simulink model "Square_PWM"  (R2019a)
settings: Solver=VariableStepAuto  StartTime=0.0  StopTime=0.2  RelTol=1e-3
libraries: powerlib x15, simulink x1, powerlib_meascontrol x1
settings Model: Creator=omar_  LastModifiedBy=omar_
settings DataIOCC: ReturnWorkspaceOutputs=off

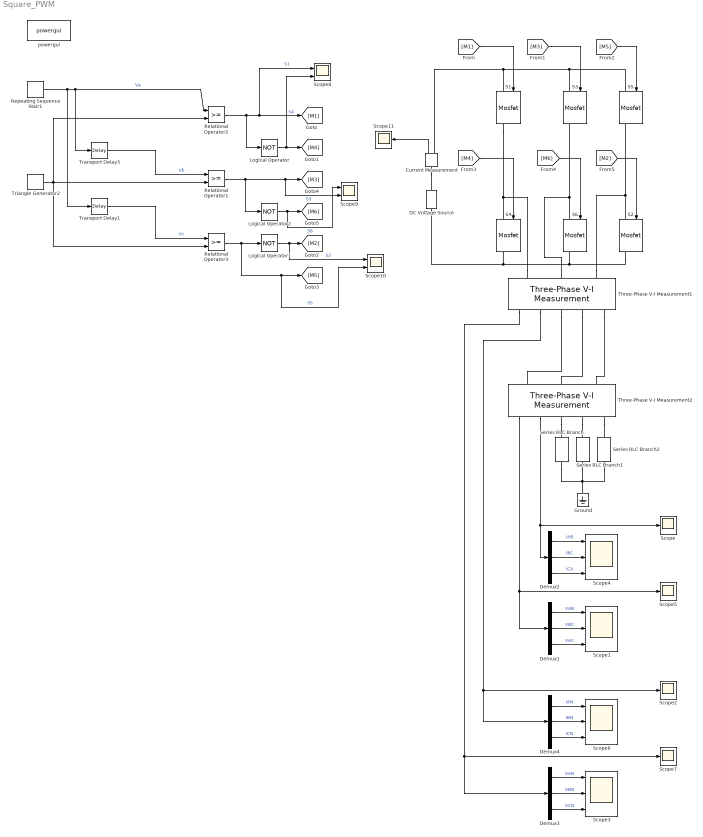
== system Square_PWM ==
  Current Measurement : powerlib/Measurements/Current Measurement  PhasorSimulation=off  OutputType=Complex  PSBequivalent=0
      settings: SourceProductName=Simscape Electrical
  DC Voltage Source : powerlib/Electrical Sources/DC Voltage Source  Amplitude=100  Measurements=None
      settings: SourceProductName=Simscape Electrical
  Demux{1..4} (4 alike) : Demux  Outputs=3
  Ground : powerlib/Elements/Ground  LConnTagsString=a
      settings: SourceProductName=Simscape Electrical
  Logical Operator : Logic  Operator=NOT  AllPortsSameDT=off  OutDataTypeStr=boolean
  Logical Operator1 : Logic  Operator=NOT  AllPortsSameDT=off  OutDataTypeStr=boolean
  Logical Operator2 : Logic  Operator=NOT  AllPortsSameDT=off  OutDataTypeStr=boolean
  Relational Operator1 : RelationalOperator  OutDataTypeStr=boolean  RndMeth=Simplest
  Relational Operator2 : RelationalOperator  OutDataTypeStr=boolean  RndMeth=Simplest
  Relational Operator3 : RelationalOperator  OutDataTypeStr=boolean  RndMeth=Simplest
  Repeating Sequence Stair1 : simulink/Sources/Repeating Sequence Stair  OutValues=[0.707, 0.707, -0.707, -0.707].'  tsamp=0.005  OutMin=[]  OutMax=[]  OutDataTypeStr=double  OutputDataTypeScalingMode=double  OutDataType=fixdt(0,8)  ConRadixGroup=Best Precision: Vector-wise  OutScaling=2^-12
  S{1..6} (6 alike) : powerlib/Power Electronics/Mosfet  Ron=0  Lon=0  Rd=0  Vfd=0  IC=0  Rs=1e5  Cs=inf  Measurements=on
      settings: SourceProductName=Simscape Electrical
  Scope{,2,5,7,11} (5 alike) : Scope
  Scope{1,3..4,6} (4 alike) : Scope  NumInputPorts=3
  Scope10 : Scope  NumInputPorts=2
  Scope8 : Scope  NumInputPorts=2
  Scope9 : Scope  NumInputPorts=2
  Series RLC Branch : powerlib/Elements/Series RLC Branch  LConnTagsString=__new0  RConnTagsString=__new0  BranchType=RL  Resistance=1  Inductance=5e-3  SetiL0=off  InitialCurrent=0  Capacitance=1e-6  Setx0=off  InitialVoltage=0  Measurements=None
      settings: SourceProductName=Simscape Electrical
  Series RLC Branch1 : powerlib/Elements/Series RLC Branch  LConnTagsString=__new0  RConnTagsString=__new0  BranchType=RL  Resistance=1  Inductance=5e-3  SetiL0=off  InitialCurrent=0  Capacitance=1e-6  Setx0=off  InitialVoltage=0  Measurements=None
      settings: SourceProductName=Simscape Electrical
  Series RLC Branch2 : powerlib/Elements/Series RLC Branch  LConnTagsString=__new0  RConnTagsString=__new0  BranchType=RL  Resistance=1  Inductance=5e-3  SetiL0=off  InitialCurrent=0  Capacitance=1e-6  Setx0=off  InitialVoltage=0  Measurements=None
      settings: SourceProductName=Simscape Electrical
  Three-Phase V-I Measurement1 : powerlib/Measurements/Three-Phase V-I Measurement  VoltageMeasurement=phase-to-ground  SetLabelV=off  LabelV=Vabc  Vpu=off  VpuLL=off  CurrentMeasurement=yes  SetLabelI=off  LabelI=Iabc  Ipu=off  Pbase=100e6  Vbase=500e3  OutputType=Complex  PhasorSimulation=off  PSBequivalent=0
      settings: SourceProductName=Simscape Electrical
  Three-Phase V-I Measurement2 : powerlib/Measurements/Three-Phase V-I Measurement  VoltageMeasurement=phase-to-phase  SetLabelV=off  LabelV=Vabc  Vpu=off  VpuLL=off  CurrentMeasurement=yes  SetLabelI=off  LabelI=Iabc  Ipu=off  Pbase=100e6  Vbase=500e3  OutputType=Complex  PhasorSimulation=off  PSBequivalent=0
      settings: SourceProductName=Simscape Electrical
  Transport Delay1 : TransportDelay  DelayTime=(240/180)*0.01
  Transport Delay3 : TransportDelay  DelayTime=(120/180)*0.01
  Triangle Generator2 : powerlib_meascontrol/Pulse & Signal Generators/Triangle Generator  Freq=17*50  Phase=270  Ts=0
      settings: SourceProductName=Simscape Electrical
  powergui : powerlib/powergui  Priority=1  SimulationMode=Continuous  SampleTime=50e-6  frequency=60  Iterations=50  frequencyindice=0  Pbase=100e6  ErrMax=1e-4  UnitsV=kV  UnitsW=MW  buscounter=0  FunctionMessages=off  echomessages=off  EnableUseOfTLC=off  CurrentSourceSwitches=off  DisableSnubberDevices=off  DisableRonSwitches=off  DisableVfSwitches=off  DisplayEquations=off  AutomaticDiscreteSolvers=off  SolverType=Tustin/Backward Euler (TBE)  Interpol=off  ExternalGateDelay=off  methode=off  Ts=100  x0status=blocks  SPID=on  SwTol=0  HookPort=off  NonlinearTolerance=0  nMaxIteration=15  ContinueOnMaxIteration=off  RestoreLinks=warning  ResistiveCurrentMeasurement=off  Frange=[0:2:500]  Ylog=off  Xlog=on  ShowGrid=off  save=off  variable=ZData  structure=Io_Line  ZoomFFT=off  StartTime=0.08  cycles=2  DisplayStyle=2  fundamental=50  FreqAxis=off  MaxFrequency=1000  frequencyindicesteady=1  RmsSteady=1  display=off
      settings: SourceProductName=Simscape Electrical
  wires:
  Demux1/1 -> Scope1/1  "VAB"
  Demux2/2 -> Scope4/2  "IBC"
  Logical Operator/1 -> Scope8/2, [M4]  "S4"
  Demux2/1 -> Scope4/1  "IAB"
  [M4] -> S4/1
  Demux1/2 -> Scope1/2  "VBC"
  [M3] -> S3/1
  [M2] -> S2/1
  [M1] -> S1/1
  [M6] -> S6/1
  Demux2/3 -> Scope4/3  "ICA"
  Demux1/3 -> Scope1/3  "VAC"
  Logical Operator2/1 -> Scope9/2, [M6]  "S6"
  [M5] -> S5/1
  Repeating Sequence Stair1/1 -> Transport Delay1/1, Transport Delay3/1, Relational Operator2/1  "Va"
  Transport Delay3/1 -> Relational Operator1/1  "Vb"
  Transport Delay1/1 -> Relational Operator3/1  "Vc"
  Triangle Generator2/1 -> Relational Operator2/2, Relational Operator1/2, Relational Operator3/2
  Relational Operator2/1 -> Logical Operator/1, Scope8/1, [M1]  "S1"
  Relational Operator1/1 -> Scope9/1, [M3], Logical Operator2/1  "S3"
  Relational Operator3/1 -> Scope10/2, [M5], Logical Operator1/1  "S5"
  Demux3/3 -> Scope3/3  "VCN"
  Demux4/2 -> Scope6/2  "IBN"
  Demux4/1 -> Scope6/1  "IAN"
  Demux3/2 -> Scope3/2  "VBN"
  Demux4/3 -> Scope6/3  "ICN"
  Demux3/1 -> Scope3/1  "VAN"
  Three-Phase V-I Measurement2/2 -> Scope/1, Demux2/1
  Three-Phase V-I Measurement2/1 -> Scope5/1, Demux1/1
  Three-Phase V-I Measurement1/2 -> Scope2/1, Demux4/1
  Three-Phase V-I Measurement1/1 -> Scope7/1, Demux3/1
  Logical Operator1/1 -> Scope10/1, [M2]  "S2"
  Current Measurement/1 -> Scope11/1
  connections:
  Three-Phase V-I Measurement1/LConn3 -- S2/LConn1 -- S5/RConn1
  S5/LConn1 -- S3/LConn1 -- Current Measurement/RConn1 -- S1/LConn1
  S3/RConn1 -- S6/LConn1 -- Three-Phase V-I Measurement1/LConn2
  DC Voltage Source/LConn1 -- S2/RConn1 -- S6/RConn1 -- S4/RConn1
  Ground/LConn1 -- Series RLC Branch/RConn1 -- Series RLC Branch2/RConn1 -- Series RLC Branch1/RConn1
  Three-Phase V-I Measurement1/LConn1 -- S1/RConn1 -- S4/LConn1
  Three-Phase V-I Measurement1/RConn1 -- Three-Phase V-I Measurement2/LConn1
  Three-Phase V-I Measurement1/RConn2 -- Three-Phase V-I Measurement2/LConn2
  Three-Phase V-I Measurement1/RConn3 -- Three-Phase V-I Measurement2/LConn3
  Three-Phase V-I Measurement2/RConn1 -- Series RLC Branch/LConn1
  Three-Phase V-I Measurement2/RConn2 -- Series RLC Branch1/LConn1
  Three-Phase V-I Measurement2/RConn3 -- Series RLC Branch2/LConn1
  Current Measurement/LConn1 -- DC Voltage Source/RConn1
